simulink model "test_matlabfcn_offline"  (R2018a)
settings: Solver=FixedStepAuto  StartTime=0.0  StopTime=16000  FixedStep=4000  RelTol=1e-3
InitFcn:
  | stop_time_as_str = get_param(gcs, 'StopTime');
  | stop_time = str2double(stop_time_as_str);
settings Model: Creator=gmb  LastModifiedBy=gmb

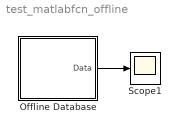
== system test_matlabfcn_offline ==
  Offline Database : Subsystem  mask{file="local.csv", date_from="2018-04-17", time_from="06:00:00", date_until="2018-04-17", time_until="10:00:00", sensors="TW,I"}
      mask prompts: date_from "Start day"; time_from "Start time"; date_until "End day"; time_until "End time"
  Scope1 : Scope
  wires:
  Offline Database/1(Data) -> Scope1/1

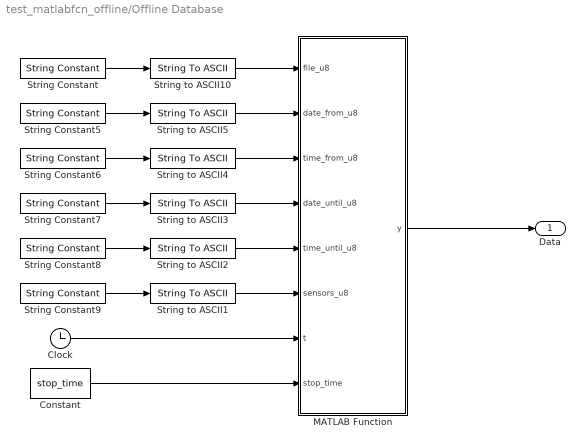
== system test_matlabfcn_offline/Offline Database ==
  Clock : Clock
  Constant : Constant  Value=stop_time
  MATLAB Function : MATLAB Function  TreatAsAtomicUnit=on
  String Constant : StringConstant  String=file
  String Constant5 : StringConstant  String=date_from
  String Constant6 : StringConstant  String=time_from
  String Constant7 : StringConstant  String=date_until
  String Constant8 : StringConstant  String=time_until
  String Constant9 : StringConstant  String=sensors
  String to ASCII{1..5,10} (6 alike) : StringToASCII
  Data : Outport
  wires:
  String to ASCII1/1 -> MATLAB Function/6(sensors_u8)
  String Constant6/1 -> String to ASCII4/1
  String Constant/1 -> String to ASCII10/1
  String Constant5/1 -> String to ASCII5/1
  String to ASCII5/1 -> MATLAB Function/2(date_from_u8)
  String to ASCII10/1 -> MATLAB Function/1(file_u8)
  String Constant9/1 -> String to ASCII1/1
  Clock/1 -> MATLAB Function/7(t)
  String to ASCII3/1 -> MATLAB Function/4(date_until_u8)
  String Constant7/1 -> String to ASCII3/1
  String to ASCII2/1 -> MATLAB Function/5(time_until_u8)
  String to ASCII4/1 -> MATLAB Function/3(time_from_u8)
  Constant/1 -> MATLAB Function/8(stop_time)
  String Constant8/1 -> String to ASCII2/1
  MATLAB Function/1(y) -> Data/1

== matlab function test_matlabfcn_offline/Offline Database/MATLAB Function ==
  data: file_u8 input; y output; date_from_u8 input; time_from_u8 input; date_until_u8 input; time_until_u8 input; sensors_u8 input; t input; stop_time input
function y = fcn(file_u8, date_from_u8, time_from_u8, date_until_u8, time_until_u8, sensors_u8, t, stop_time)

persistent init;

coder.extrinsic('fullfile', 'loadlibrary', 'system_dependent', 'libfunctions','calllib','unloadlibrary', 'libpointer', 'resolve_pointer');

incpath = fullfile('c:\Program Files\','MySQL','MySQL Connector C 6.1','include');
[~, ~] = loadlibrary(['simdatabase',system_dependent('GetSharedLibExt')],'simdatabase.h', 'includepath', incpath);

if isempty(init)
   calllib('simdatabase','simdatabase_init');
   init = 1;
end

file = char(file_u8);
date_from = char(date_from_u8);
time_from = char(time_from_u8);
date_until = char(date_until_u8);
time_until = char(time_until_u8);
sensors = char(sensors_u8);

vals = zeros(1, 10);
valPtr = libpointer('doublePtr', vals);
y = zeros(1, 10);

calllib('simdatabase','simdatabase_step_local', file, date_from, time_from, date_until, time_until, sensors, t, valPtr);

if(t >= stop_time)
   calllib('simdatabase','simdatabase_term');
   unloadlibrary('simdatabase');
end

y = resolve_pointer(valPtr);
